simulink model "HW02_Tirel_Sim1_Mot"  (R2020b)
settings: Solver=VariableStepAuto  StartTime=0.0  StopTime=1  RelTol=1e-3
values from neighbouring files (symbols this model uses):
  Bm = 1.02*10^-9    (= 1.02e-09)    [HW02_Tirel_Mat_Mot.m]
  Jm = 9.5*10^-10    (= 9.5e-10)    [HW02_Tirel_Mat_Mot.m]
  ke = 0.000114    [HW02_Tirel_Mat_Mot.m]
  km = 0.00109    [HW02_Tirel_Mat_Mot.m]
  La = 28*10^-6    (= 2.8e-05)    [HW02_Tirel_Mat_Mot.m]
  Ra = 8.8    [HW02_Tirel_Mat_Mot.m]
  Tl = MTl/2    (= 0.000366)    [HW02_Tirel_Mat_Mot.m]
  Ts = 0.000011    (= 1.1e-05)    [HW02_Tirel_Mat_Mot.m]
undefined symbols (not defined in the file or in its folder): Kn, Kn1
libraries: cstblocks x3, simulink x3
settings Model: Creator=DELL  LastModifiedBy=DELL

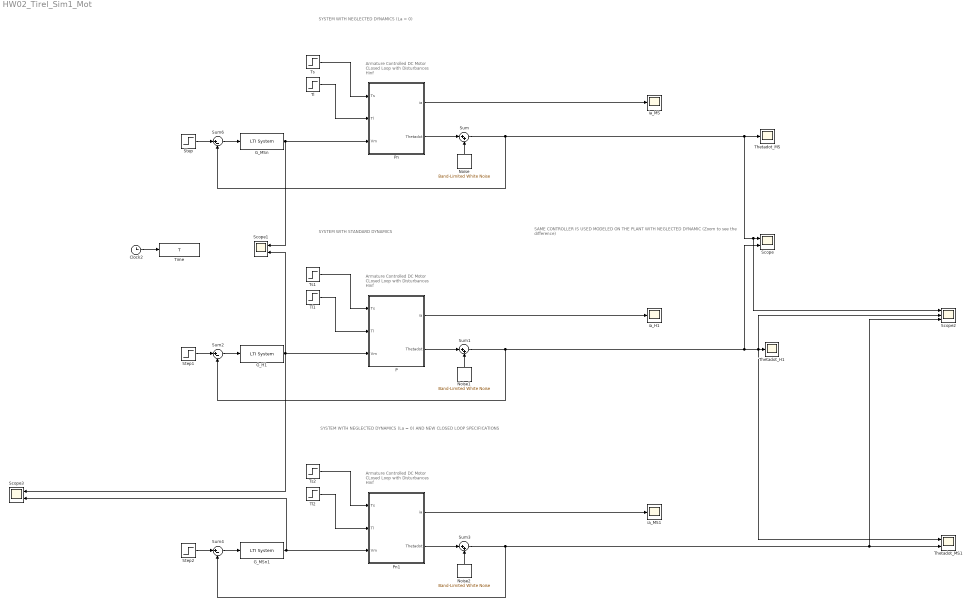
== system HW02_Tirel_Sim1_Mot ==
  note: SAME CONTROLLER IS USED MODELED ON THE PLANT WITH NEGLECTED DYNAMIC
      | (Zoom to see the difference)
  note: Armature Controlled DC Motor
      | CLosed Loop with Disturbances Hinf
  note: SYSTEM WITH NEGLECTED DYNAMICS (La = 0)
  note: Armature Controlled DC Motor
      | CLosed Loop with Disturbances Hinf
  note: SYSTEM WITH STANDARD DYNAMICS
  note: Armature Controlled DC Motor
      | CLosed Loop with Disturbances Hinf
  note: SYSTEM WITH NEGLECTED DYNAMICS (La = 0) AND NEW CLOSED LOOP SPECIFICATIONS
  Clock2 : Clock
  G_H1 : cstblocks/LTI System  sys=tf(Kn)  IC=[]
  G_MSn : cstblocks/LTI System  sys=tf(Kn)  IC=[]
  G_MSn1 : cstblocks/LTI System  sys=tf(Kn1)  IC=[]
  Noise : simulink/Sources/Band-Limited White Noise  Cov=[0.001]  Ts=0.001  seed=[23341]
  Noise1 : simulink/Sources/Band-Limited White Noise  Cov=[0.001]  Ts=0.001  seed=[23341]
  Noise2 : simulink/Sources/Band-Limited White Noise  Cov=[0.001]  Ts=0.001  seed=[23341]
  P : Subsystem
  Pn : Subsystem
  Pn1 : Subsystem
  Scope : Scope  NumInputPorts=2
  Scope1 : Scope  NumInputPorts=2
  Scope2 : Scope  NumInputPorts=3
  Scope3 : Scope  NumInputPorts=2
  Step : Step  Time=0  After=25000  SampleTime=0
  Step1 : Step  Time=0  After=25000  SampleTime=0
  Step2 : Step  Time=0  After=25000  SampleTime=0
  Sum : Sum  Inputs=|++
  Sum1 : Sum  Inputs=|++
  Sum2 : Sum  Inputs=|+-
  Sum3 : Sum  Inputs=|++
  Sum4 : Sum  Inputs=|+-
  Sum6 : Sum  Inputs=|+-
  Thetadot_H1 : Scope
  Thetadot_MS : Scope
  Thetadot_MS1 : Scope  NumInputPorts=2
  Time : ToWorkspace  VariableName=T  SaveFormat=Timeseries  SampleTime=-1
  Tl : Step  Time=0.5  After=Tl  SampleTime=0
  Tl1 : Step  Time=0.5  After=Tl  SampleTime=0
  Tl2 : Step  Time=0.5  After=Tl  SampleTime=0
  Ts : Step  Time=0  After=Ts  SampleTime=0
  Ts1 : Step  Time=0  After=Ts  SampleTime=0
  Ts2 : Step  Time=0  After=Ts  SampleTime=0
  ia_H1 : Scope
  ia_MS : Scope
  ia_MS1 : Scope
  wires:
  Sum6/1 -> G_MSn/1
  Pn/2(Thetadot) -> Sum/1
  Sum/1 -> Sum6/2, Thetadot_MS/1, Scope2/1, Scope/1
  Noise/1 -> Sum/2
  G_MSn/1 -> Scope1/1, Pn/3(Vm)
  Pn/1(ia) -> ia_MS/1
  Ts/1 -> Pn/1(Ts)
  Tl/1 -> Pn/2(Tl)
  Sum2/1 -> G_H1/1
  P/2(Thetadot) -> Sum1/1
  Sum1/1 -> Sum2/2, Thetadot_MS1/1, Thetadot_H1/1, Scope2/2, Scope/2
  Noise1/1 -> Sum1/2
  G_H1/1 -> Scope3/1, Scope1/2, P/3(Vm)
  P/1(ia) -> ia_H1/1
  Ts1/1 -> P/1(Ts)
  Tl1/1 -> P/2(Tl)
  Clock2/1 -> Time/1
  Step/1 -> Sum6/1
  Step1/1 -> Sum2/1
  Pn1/2(Thetadot) -> Sum3/1
  Sum4/1 -> G_MSn1/1
  Sum3/1 -> Sum4/2, Scope2/3, Thetadot_MS1/2
  Ts2/1 -> Pn1/1(Ts)
  G_MSn1/1 -> Scope3/2, Pn1/3(Vm)
  Tl2/1 -> Pn1/2(Tl)
  Pn1/1(ia) -> ia_MS1/1
  Step2/1 -> Sum4/1
  Noise2/1 -> Sum3/2

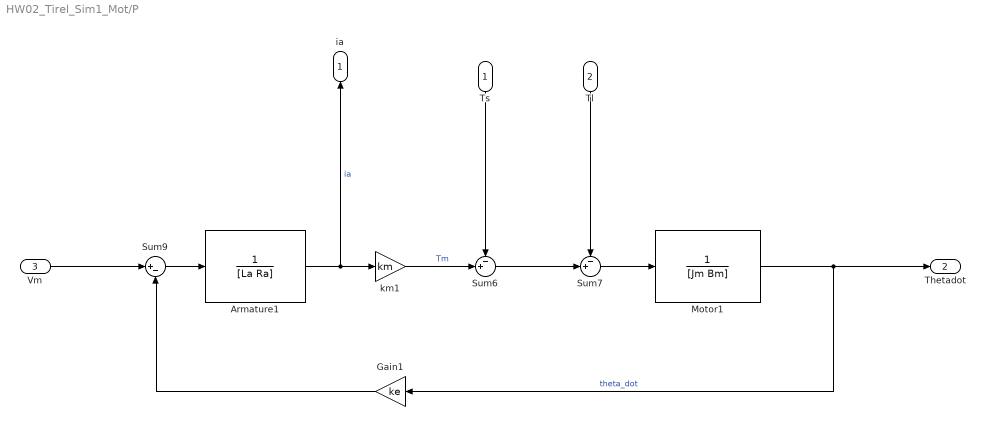
== system HW02_Tirel_Sim1_Mot/P ==
  Ts : Inport
  Tl : Inport  Port=2
  Vm : Inport  Port=3
  Armature1 : TransferFcn  Denominator=[La Ra]
  Gain1 : Gain  Gain=ke
  Motor1 : TransferFcn  Denominator=[Jm Bm]
  Sum6 : Sum  Inputs=-+|
  Sum7 : Sum  Inputs=-+|
  Sum9 : Sum  Inputs=|+-
  km1 : Gain  Gain=km
  ia : Outport
  Thetadot : Outport  Port=2
  wires:
  Sum9/1 -> Armature1/1
  Gain1/1 -> Sum9/2
  Armature1/1 -> ia/1, km1/1  "ia"
  Motor1/1 -> Thetadot/1, Gain1/1  "theta_dot"
  Sum6/1 -> Sum7/2
  Sum7/1 -> Motor1/1
  Tl/1 -> Sum7/1
  km1/1 -> Sum6/2  "Tm"
  Vm/1 -> Sum9/1
  Ts/1 -> Sum6/1

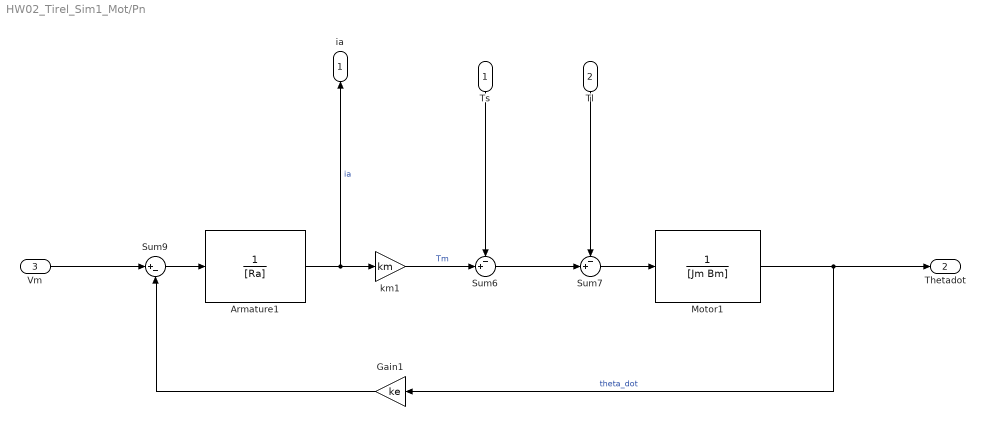
== system HW02_Tirel_Sim1_Mot/Pn ==
  Ts : Inport
  Tl : Inport  Port=2
  Vm : Inport  Port=3
  Armature1 : TransferFcn  Denominator=[Ra]
  Gain1 : Gain  Gain=ke
  Motor1 : TransferFcn  Denominator=[Jm Bm]
  Sum6 : Sum  Inputs=-+|
  Sum7 : Sum  Inputs=-+|
  Sum9 : Sum  Inputs=|+-
  km1 : Gain  Gain=km
  ia : Outport
  Thetadot : Outport  Port=2
  wires:
  Sum9/1 -> Armature1/1
  Gain1/1 -> Sum9/2
  Armature1/1 -> ia/1, km1/1  "ia"
  Motor1/1 -> Thetadot/1, Gain1/1  "theta_dot"
  Sum6/1 -> Sum7/2
  Sum7/1 -> Motor1/1
  Tl/1 -> Sum7/1
  km1/1 -> Sum6/2  "Tm"
  Vm/1 -> Sum9/1
  Ts/1 -> Sum6/1

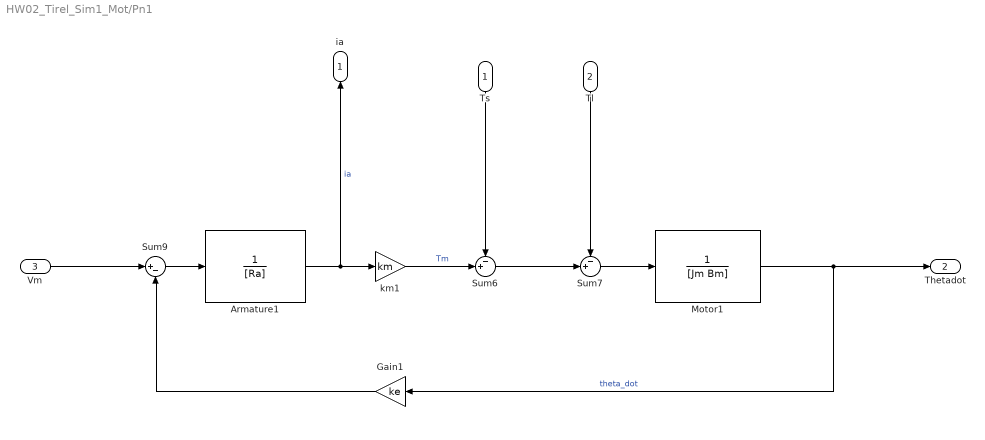
== system HW02_Tirel_Sim1_Mot/Pn1 ==
  Ts : Inport
  Tl : Inport  Port=2
  Vm : Inport  Port=3
  Armature1 : TransferFcn  Denominator=[Ra]
  Gain1 : Gain  Gain=ke
  Motor1 : TransferFcn  Denominator=[Jm Bm]
  Sum6 : Sum  Inputs=-+|
  Sum7 : Sum  Inputs=-+|
  Sum9 : Sum  Inputs=|+-
  km1 : Gain  Gain=km
  ia : Outport
  Thetadot : Outport  Port=2
  wires:
  Sum9/1 -> Armature1/1
  Gain1/1 -> Sum9/2
  Armature1/1 -> ia/1, km1/1  "ia"
  Motor1/1 -> Thetadot/1, Gain1/1  "theta_dot"
  Sum6/1 -> Sum7/2
  Sum7/1 -> Motor1/1
  Tl/1 -> Sum7/1
  km1/1 -> Sum6/2  "Tm"
  Vm/1 -> Sum9/1
  Ts/1 -> Sum6/1
